simulink model "siasun_config_casadi_VS_lsj_robot_16a"  (R2020a)
settings: Solver=FixedStepAuto  StartTime=0.0  StopTime=inf  FixedStep=0.001  RelTol=1e-3  EnableMultiTasking=on
libraries: Robot_ToolBox x20
(part 1 of 6)
settings Model: SimulationMode=external  Creator=Wang Yifan  LastModifiedBy=admin
settings DataIOCC: ReturnWorkspaceOutputs=off
settings OptimizationCC: LifeSpan=Inf  EfficientTunableParamExpr=on
settings DebuggingCC: SFUnexpectedBacktrackingDiag=warning  SFNoUnconditionalDefaultTransitionDiag=warning  ArithmeticOperatorsInVariantConditions=warning
settings HardwareCC: ProdBitPerLong=64  ProdHWDeviceType=Intel->x86-64 (Linux 64)  TargetBitPerLong=64  TargetBitPerPointer=64  TargetBitPerSizeT=64  TargetBitPerPtrDiffT=64  TargetLargestAtomicFloat=Float  TargetIntDivRoundTo=Zero  TargetEndianess=LittleEndian  TargetWordSize=64  TargetHWDeviceType=Intel->x86-64 (Linux 64)  ProdEqTarget=off
settings SFSimCC: SimUseLocalCustomCode=off  MATLABDynamicMemAlloc=off  CustomCodeUndefinedFunction=UseInterfaceOnly
settings RTWCC: Description=Linux Embedded Real-Time target  SystemTargetFile=linux_ert_target.tlc  GenCodeOnly=on  MakeCommand=make_rtw CC=gcc  TemplateMakefile=linux_ert_target.tmf  RetainRTWFile=on  RTWUseLocalCustomCode=off
settings CodeAppCC: ForceParamTrailComments=on  IgnoreCustomStorageClasses=off  OperatorAnnotations=on  SimulinkDataObjDesc=on  SFDataObjDesc=on  MATLABFcnDesc=on  InsertBlockDesc=on  StateflowObjectComments=on  MATLABSourceComments=on
settings STFCustomTargetCC: CombineOutputUpdateFcns=on  ERTCustomFileBanners=on  SupportContinuousTime=off  SupportNonInlinedSFcns=off  RemoveResetFunc=on  MATLABClassNameForMDSCustomization=Simulink.SoftwareTarget.ERTCustomization  SystemTargetFile=linux_ert_target.tlc
settings ERTTargetCC: MultiwordLength=2048  ParMdlRefBuildCompliant=off  CompOptLevelCompliant=off  ConcurrentExecutionCompliant=off  ModelStepFunctionPrototypeControlCompliant=off  CPPClassGenCompliant=off  UseToolchainInfoCompliant=off  ExtMode=on  ExtModeMexArgs='192.168.0.99' 1 17725  ERTSrcFileBannerTemplate=linux_ert_target_code_template.cgt  ERTHdrFileBannerTemplate=linux_ert_target_code_template.cgt  ERTDataSrcFileTemplate=linux_ert_target_code_template.cgt  ERTDataHdrFileTemplate=linux_ert_target_code_template.cgt  ERTCustomFileTemplate=linux_ert_target_generate_main.tlc
settings ConfigComp: CovMetricSettings=dw  CovSaveCumulativeToWorkspaceVar=on  CovSaveSingleToWorkspaceVar=on  CovExternalEMLEnable=off

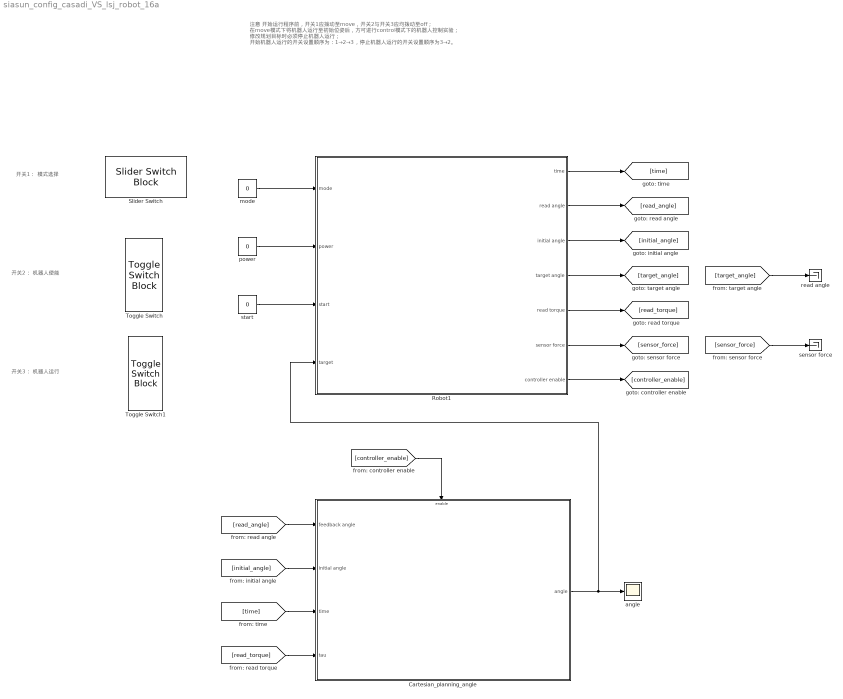
== system siasun_config_casadi_VS_lsj_robot_16a ==
  note: 开关3： 机器人运行
  note: 开关1： 模式选择
  note: 开关2： 机器人使能
  note: 注意
      |
      | 开始运行程序前，开关1应拨动至move，开关2与开关3应均拨动至off；
      | 在move模式下将机器人运行至初始位姿后，方可进行control模式下的机器人控制实验；
      | 修改规划目标时必须停止机器人运行；
      | 开始机器人运行的开关设置顺序为：1→2→3，停止机器人运行的开关设置顺序为3→2。
  Cartesian_planning_angle : Subsystem
  Robot1 : Subsystem  mask{move_joint=[0 0 0 0 0 0], joint_1_limit=[-pi*0.94, pi*0.94], joint_2_limit=[-pi/2, pi*0.72], joint_3_limit=[-pi*0.94, pi*0.42], joint_4_limit=[-pi/1, pi/1], joint_5_limit=[-pi*0.67, pi*0.67], joint_6_limit=[-pi/0.5, pi/0.5]}
      mask prompts: joint_1_limit "Joint 1"; joint_2_limit "Joint 2"; joint_3_limit "Joint 3"; joint_4_limit "Joint 4"; joint_5_limit "Joint 5"; joint_6_limit "Joint 6"
      mask DialogControl Container1 Prompt: 目标关节角(rad)
      mask DialogControl Control1 Prompt: e.g. [0 0 0 0 0 0]
      mask DialogControl Container2 Prompt: 关节限位(rad)
      mask DialogControl Control2 Prompt: e.g. [-pi/2, pi/2]
      mask DialogControl Container3 Prompt: 注意：不需要对此模块内部进行修改
  Slider Switch : SliderSwitchBlock  LabelPosition=Hide
      settings: Values={{'control', 'move'}, [0 1]}
  Toggle Switch : ToggleSwitchBlock  LabelPosition=Hide
      settings: Values={{'Off', 'On'}, [0 1]}
  Toggle Switch1 : ToggleSwitchBlock  LabelPosition=Hide
      settings: Values={{'Off', 'On'}, [0 1]}
  angle : Scope
  mode : Constant  Value=0
  power : Constant  Value=0
  read angle : Terminator
  sensor force : Terminator
  start : Constant  Value=0
  wires:
  mode/1 -> Robot1/1(mode)
  power/1 -> Robot1/2(power)
  Robot1/2(read angle) -> [read_angle]
  Robot1/1(time) -> [time]
  Robot1/7(controller enable) -> [controller_enable]
  Robot1/4(target angle) -> [target_angle]
  Robot1/6(sensor force) -> [sensor_force]
  Robot1/3(initial angle) -> [initial_angle]
  Robot1/5(read torque) -> [read_torque]
  [read_torque] -> Cartesian_planning_angle/4(tau)
  [sensor_force] -> sensor force/1
  start/1 -> Robot1/3(start)
  Cartesian_planning_angle/1(angle) -> angle/1, Robot1/4(target)
  [controller_enable] -> Cartesian_planning_angle/Enable
  [initial_angle] -> Cartesian_planning_angle/2(initial angle)
  [time] -> Cartesian_planning_angle/3(time)
  [read_angle] -> Cartesian_planning_angle/1(feedback angle)
  [target_angle] -> read angle/1

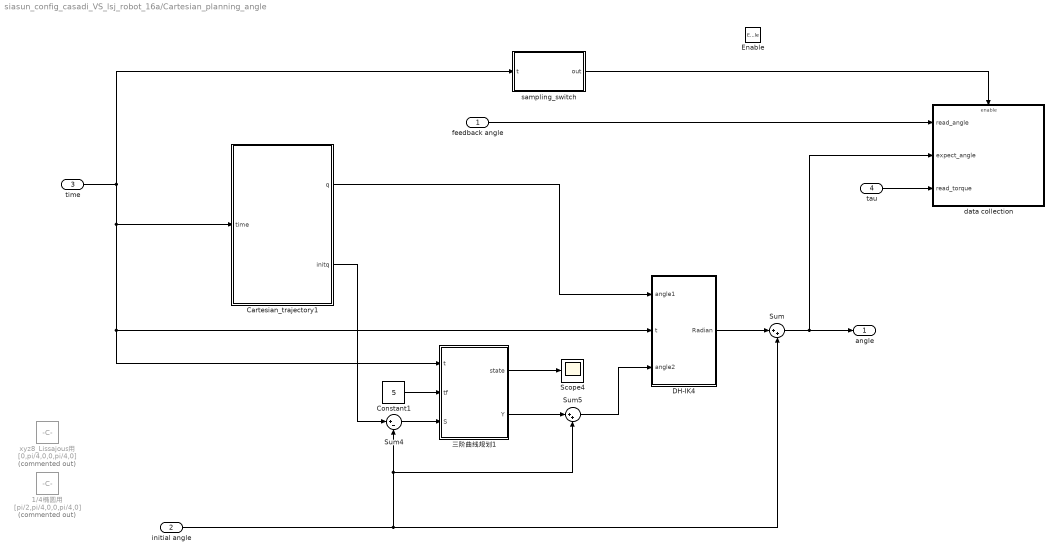
== system siasun_config_casadi_VS_lsj_robot_16a/Cartesian_planning_angle ==
  feedback angle : Inport
  initial angle : Inport  Port=2
  time : Inport  Port=3
  tau : Inport  Port=4
  Enable : EnablePort
  1/4椭圆用 : Constant  Commented=on  Value=[pi/2,pi/4,0,0,pi/4,0]
  Cartesian_trajectory1 : MATLAB Function  TreatAsAtomicUnit=on
  Constant1 : Constant  Value=5
  DH-IK4 : MATLAB Function  TreatAsAtomicUnit=on
  Scope4 : Scope
  Sum : Sum  Inputs=|++
  Sum4 : Sum  Inputs=|+-
  Sum5 : Sum  Inputs=|++
  data collection : Subsystem
  sampling_switch : MATLAB Function  TreatAsAtomicUnit=on
  xyz8_Lissajous用 : Constant  Commented=on  Value=[0,pi/4,0,0,pi/4,0]
  三阶曲线规划1 : Subsystem
  angle : Outport
  wires:
  DH-IK4/1(Radian) -> Sum/1
  Cartesian_trajectory1/1(q) -> DH-IK4/1(angle1)
  initial angle/1 -> Sum5/2, Sum4/2, Sum/2
  Sum4/1 -> 三阶曲线规划1/3(S)
  Constant1/1 -> 三阶曲线规划1/2(tf)
  三阶曲线规划1/1(state) -> Scope4/1
  三阶曲线规划1/2(Y) -> Sum5/1
  Sum5/1 -> DH-IK4/3(angle2)
  sampling_switch/1(out) -> data collection/Enable
  feedback angle/1 -> data collection/1(read_angle)
  Sum/1 -> angle/1, data collection/2(expect_angle)
  time/1 -> DH-IK4/2(t), 三阶曲线规划1/1(t), Cartesian_trajectory1/1(time), sampling_switch/1(t)
  tau/1 -> data collection/3(read_torque)
  Cartesian_trajectory1/2(initq) -> Sum4/1

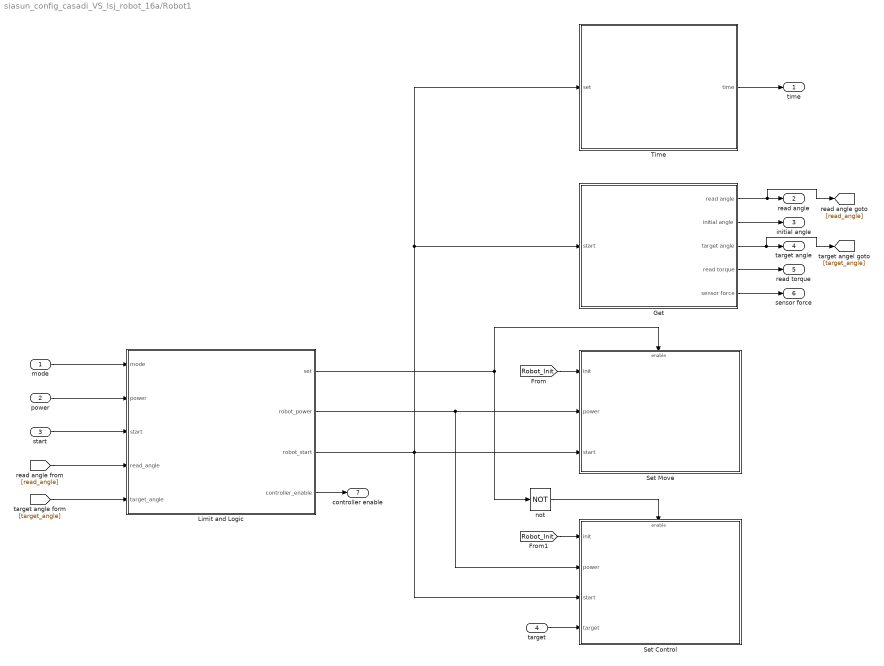
== system siasun_config_casadi_VS_lsj_robot_16a/Robot1 ==
  mode : Inport
  power : Inport  Port=2
  start : Inport  Port=3
  target : Inport  Port=4
  Get : Subsystem
  Limit and Logic : Subsystem
  Set Control : Subsystem  mask(机器人控制模式){mode=Position Mode}
      mask prompts: mode "Control Mode"
      mask TypeOptions mode: Position Mode | Torque Mode | Velocity Mode
  Set Move : Subsystem
  Time : Subsystem
  not : Logic  Operator=NOT  AllPortsSameDT=off  OutDataTypeStr=boolean
  time : Outport
  read angle : Outport  Port=2
  initial angle : Outport  Port=3
  target angle : Outport  Port=4
  read torque : Outport  Port=5
  sensor force : Outport  Port=6
  controller enable : Outport  Port=7
  wires:
  target/1 -> Set Control/4(target)
  Get/1(read angle) -> [read_angle], read angle/1
  Time/1(time) -> time/1
  Get/2(initial angle) -> initial angle/1
  Get/3(target angle) -> [target_angle], target angle/1
  Get/5(sensor force) -> sensor force/1
  Limit and Logic/1(set) -> Set Move/Enable, not/1
  not/1 -> Set Control/Enable
  Limit and Logic/2(robot_power) -> Set Control/2(power), Set Move/2(power)
  Limit and Logic/4(controller_enable) -> controller enable/1
  Limit and Logic/3(robot_start) -> Set Control/3(start), Set Move/3(start), Time/1(set), Get/1(start)
  [Robot_Init] -> Set Move/1(init)
  [Robot_Init] -> Set Control/1(init)
  Get/4(read torque) -> read torque/1
  mode/1 -> Limit and Logic/1(mode)
  power/1 -> Limit and Logic/2(power)
  start/1 -> Limit and Logic/3(start)
  [read_angle] -> Limit and Logic/4(read_angle)
  [target_angle] -> Limit and Logic/5(target_angle)

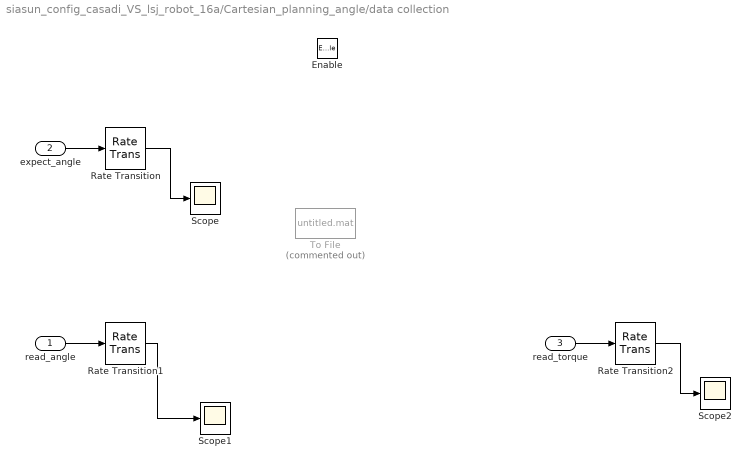
== system siasun_config_casadi_VS_lsj_robot_16a/Cartesian_planning_angle/data collection ==
  read_angle : Inport
  expect_angle : Inport  Port=2
  read_torque : Inport  Port=3
  Enable : EnablePort
  Rate Transition : RateTransition
  Rate Transition1 : RateTransition
  Rate Transition2 : RateTransition
  Scope : Scope
  Scope1 : Scope
  Scope2 : Scope
  To File : ToFile  Commented=on  SaveFormat=Timeseries
  wires:
  Rate Transition/1 -> Scope/1
  Rate Transition1/1 -> Scope1/1
  expect_angle/1 -> Rate Transition/1
  read_angle/1 -> Rate Transition1/1
  Rate Transition2/1 -> Scope2/1
  read_torque/1 -> Rate Transition2/1

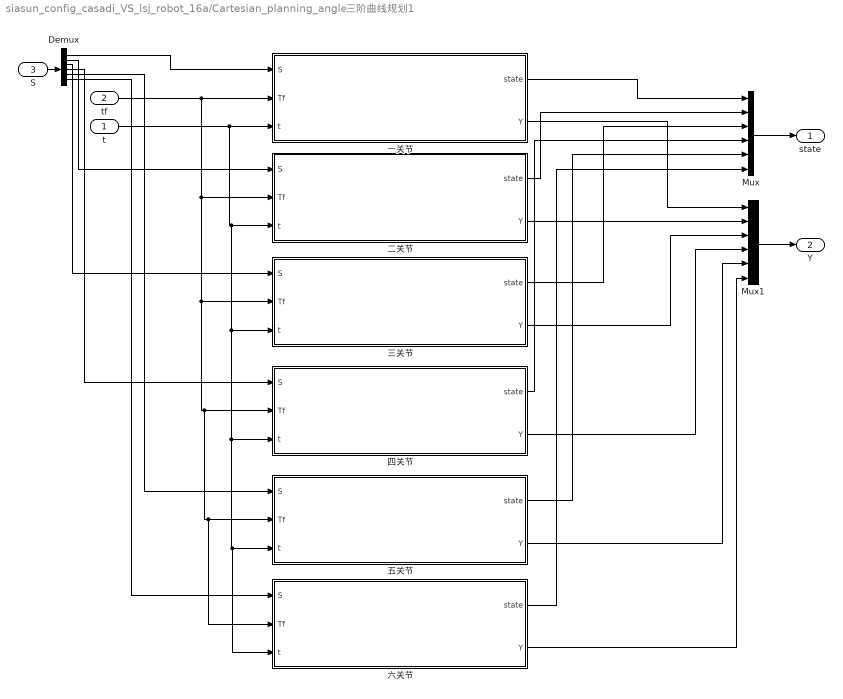
== system siasun_config_casadi_VS_lsj_robot_16a/Cartesian_planning_angle/三阶曲线规划1 ==
  t : Inport
  tf : Inport  Port=2
  S : Inport  Port=3
  Demux : Demux  Outputs=6
  Mux : Mux  Inputs=6
  Mux1 : Mux  Inputs=6
  一关节 : Subsystem
  三关节 : Subsystem
  二关节 : Subsystem
  五关节 : Subsystem
  六关节 : Subsystem
  四关节 : Subsystem
  state : Outport
  Y : Outport  Port=2
  wires:
  一关节/2(Y) -> Mux1/1
  tf/1 -> 六关节/2(Tf), 五关节/2(Tf), 四关节/2(Tf), 三关节/2(Tf), 二关节/2(Tf), 一关节/2(Tf)
  t/1 -> 六关节/3(t), 五关节/3(t), 四关节/3(t), 三关节/3(t), 二关节/3(t), 一关节/3(t)
  一关节/1(state) -> Mux/1
  三关节/1(state) -> Mux/3
  二关节/1(state) -> Mux/2
  四关节/1(state) -> Mux/4
  S/1 -> Demux/1
  Demux/1 -> 一关节/1(S)
  Demux/2 -> 二关节/1(S)
  Demux/3 -> 三关节/1(S)
  Demux/4 -> 四关节/1(S)
  Demux/5 -> 五关节/1(S)
  Demux/6 -> 六关节/1(S)
  Mux1/1 -> Y/1
  二关节/2(Y) -> Mux1/2
  三关节/2(Y) -> Mux1/3
  四关节/2(Y) -> Mux1/4
  五关节/2(Y) -> Mux1/5
  六关节/2(Y) -> Mux1/6
  Mux/1 -> state/1
  五关节/1(state) -> Mux/5
  六关节/1(state) -> Mux/6

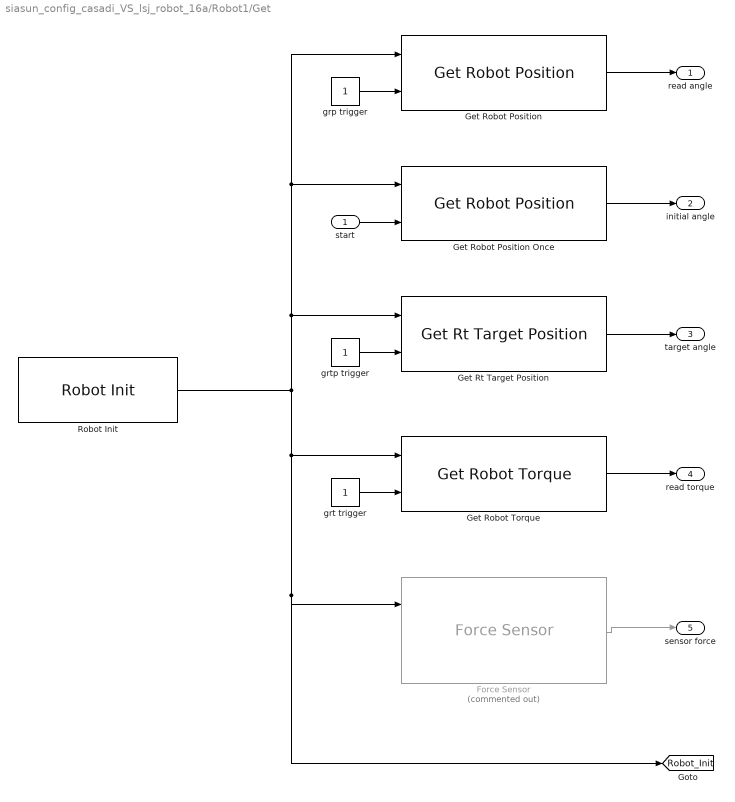
== system siasun_config_casadi_VS_lsj_robot_16a/Robot1/Get ==
  start : Inport
  Force Sensor : Robot_ToolBox/Sensor/Force Sensor  Commented=on  p_robot_index=0  p_torsensor_index=0  p_tool=0  p_wobj=0  p_transform_flag=on
  Get Robot Position : Robot_ToolBox/Robot Interface/Get Robot Position  p_robot_index=0  p_block_index=1  p_read_once=off
  Get Robot Position Once : Robot_ToolBox/Robot Interface/Get Robot Position  p_robot_index=0  p_block_index=0  p_read_once=on
  Get Robot Torque : Robot_ToolBox/Robot Interface/Get Robot Torque  p_robot_index=0  p_block_index=0  p_read_once=off
  Get Rt Target Position : Robot_ToolBox/Robot Interface/Get Rt Target Position  p_robot_index=0  p_block_index=0  p_read_once=off
  Robot Init : Robot_ToolBox/Robot System Tool/Robot Init
  grp trigger : Constant
  grt trigger : Constant
  grtp trigger : Constant
  read angle : Outport
  initial angle : Outport  Port=2
  target angle : Outport  Port=3
  read torque : Outport  Port=4
  sensor force : Outport  Port=5
  tag scope: Robot_Init=global
  wires:
  Robot Init/1 -> Get Robot Position/1, Get Robot Position Once/1, Get Rt Target Position/1, [Robot_Init], Force Sensor/1, Get Robot Torque/1
  Get Robot Position/1 -> read angle/1
  Get Robot Position Once/1 -> initial angle/1
  Get Rt Target Position/1 -> target angle/1
  Force Sensor/1 -> sensor force/1
  grp trigger/1 -> Get Robot Position/2
  grtp trigger/1 -> Get Rt Target Position/2
  start/1 -> Get Robot Position Once/2
  grt trigger/1 -> Get Robot Torque/2
  Get Robot Torque/1 -> read torque/1

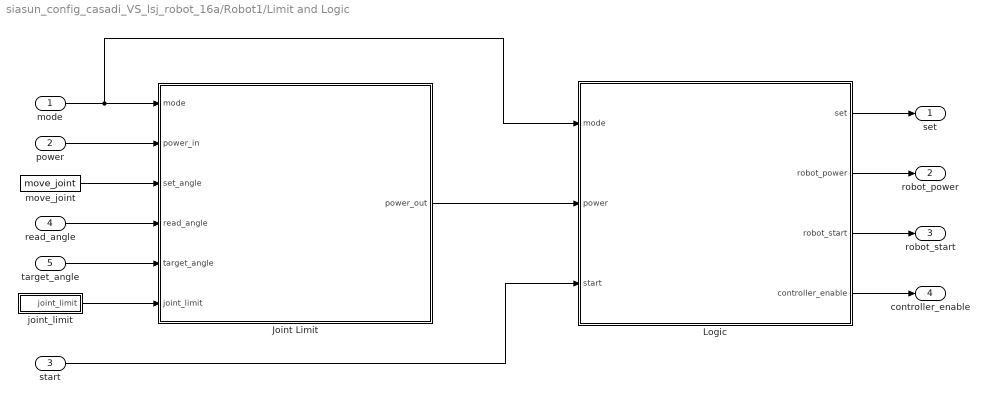
== system siasun_config_casadi_VS_lsj_robot_16a/Robot1/Limit and Logic ==
  mode : Inport
  power : Inport  Port=2
  start : Inport  Port=3
  read_angle : Inport  Port=4
  target_angle : Inport  Port=5
  Joint Limit : MATLAB Function  TreatAsAtomicUnit=on
  Logic : Stateflow chart  TreatAsAtomicUnit=on
  joint_limit : Subsystem
  move_joint : Constant  Value=move_joint
  set : Outport
  robot_power : Outport  Port=2
  robot_start : Outport  Port=3
  controller_enable : Outport  Port=4
  wires:
  Joint Limit/1(power_out) -> Logic/2(power)
  read_angle/1 -> Joint Limit/4(read_angle)
  target_angle/1 -> Joint Limit/5(target_angle)
  mode/1 -> Logic/1(mode), Joint Limit/1(mode)
  power/1 -> Joint Limit/2(power_in)
  start/1 -> Logic/3(start)
  Logic/1(set) -> set/1
  Logic/2(robot_power) -> robot_power/1
  Logic/3(robot_start) -> robot_start/1
  Logic/4(controller_enable) -> controller_enable/1
  move_joint/1 -> Joint Limit/3(set_angle)
  joint_limit/1(joint_limit) -> Joint Limit/6(joint_limit)

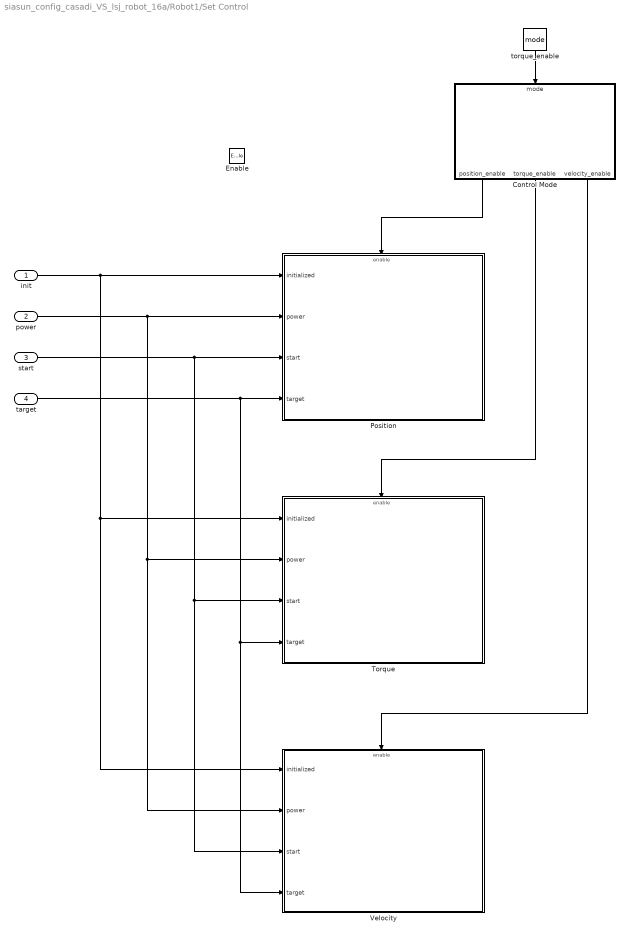
== system siasun_config_casadi_VS_lsj_robot_16a/Robot1/Set Control ==
  init : Inport
  power : Inport  Port=2
  start : Inport  Port=3
  target : Inport  Port=4
  Enable : EnablePort
  Control Mode : Stateflow chart  TreatAsAtomicUnit=on
  Position : Subsystem
  Torque : Subsystem
  Velocity : Subsystem
  torque_enable : Constant  Value=mode
  wires:
  init/1 -> Position/1(initialized), Velocity/1(initialized), Torque/1(initialized)
  power/1 -> Velocity/2(power), Torque/2(power), Position/2(power)
  start/1 -> Velocity/3(start), Torque/3(start), Position/3(start)
  target/1 -> Velocity/4(target), Torque/4(target), Position/4(target)
  Control Mode/1(position_enable) -> Position/Enable
  torque_enable/1 -> Control Mode/1(mode)
  Control Mode/2(torque_enable) -> Torque/Enable
  Control Mode/3(velocity_enable) -> Velocity/Enable

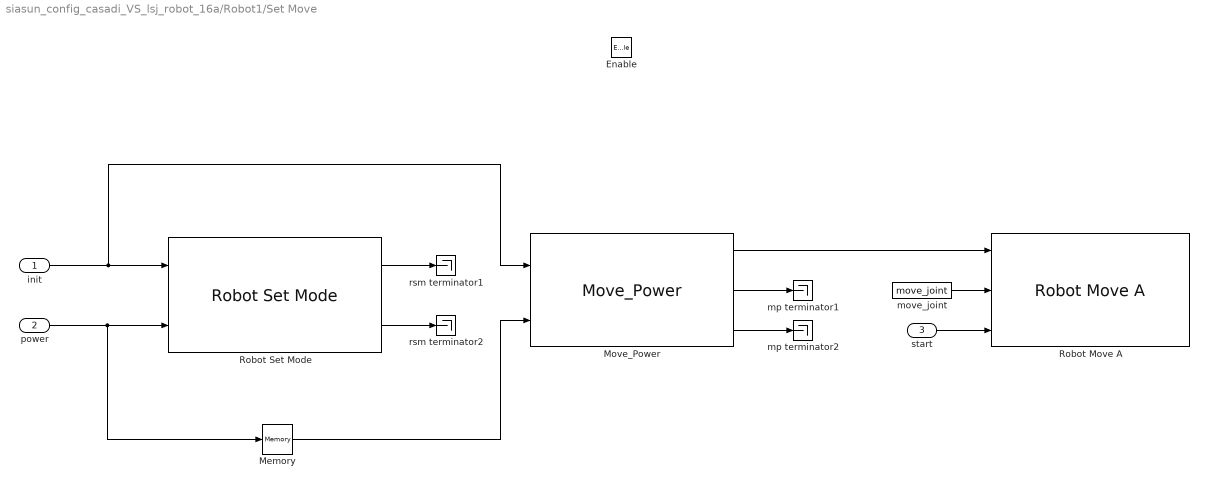
== system siasun_config_casadi_VS_lsj_robot_16a/Robot1/Set Move ==
  init : Inport
  power : Inport  Port=2
  start : Inport  Port=3
  Enable : EnablePort
  Memory : Memory
  Move_Power : Robot_ToolBox/Robot Base Conrtrol/Move_Power  p_robot_index=0  p_block_index=0
      link override S-Function Builder: Parameters=p_robot_index,p_block_index,p_move_thread
  Robot Move A : Robot_ToolBox/Robot Base Conrtrol/Robot Move A  p_robot_index=0  p_block_index=0  p_MoveA_per=[10 10 10 10 10 10]  p_MoveA_per_flag=2  p_zone=0  p_tool=0  p_wobj=0
      link override MoveA: Parameters=p_robot_index,p_block_index,p_MoveA_per,int32(p_MoveA_per_flag),p_zone,p_tool,p_wobj
  Robot Set Mode : Robot_ToolBox/Robot System Tool/Robot Set Mode  p_robot_index=0  p_block_index=0  p_robot_mode=位置模式  p_robot_all=on  p_robot_Axis1=on  p_robot_Axis2=on  p_robot_Axis3=on  p_robot_Axis4=on  p_robot_Axis5=on  p_robot_Axis6=on  p_robot_Axis_add=off
  move_joint : Constant  Value=move_joint
  mp terminator1 : Terminator
  mp terminator2 : Terminator
  rsm terminator1 : Terminator
  rsm terminator2 : Terminator
  wires:
  Move_Power/1 -> Robot Move A/1
  move_joint/1 -> Robot Move A/2
  Move_Power/2 -> mp terminator1/1
  Move_Power/3 -> mp terminator2/1
  start/1 -> Robot Move A/3
  power/1 -> Robot Set Mode/2, Memory/1
  Robot Set Mode/1 -> rsm terminator1/1
  Memory/1 -> Move_Power/2
  Robot Set Mode/2 -> rsm terminator2/1
  init/1 -> Move_Power/1, Robot Set Mode/1

== system siasun_config_casadi_VS_lsj_robot_16a/Robot1/Time ==
  set : Inport
  MATLAB Function : MATLAB Function  TreatAsAtomicUnit=on
  Memory : Memory
  time : Outport
  wires:
  set/1 -> MATLAB Function/1(set)
  MATLAB Function/1(t_out) -> time/1, Memory/1
  Memory/1 -> MATLAB Function/2(t_in)

== system siasun_config_casadi_VS_lsj_robot_16a/Cartesian_planning_angle/三阶曲线规划1/一关节 ==
  S : Inport
  Tf : Inport  Port=2
  t : Inport  Port=3
  3_planning1 : MATLAB Function  TreatAsAtomicUnit=on  mask{g_vs=0, g_ve=0}
      mask prompts: g_vs "初始速度"; g_ve "末速度"
  Interpolation3 : MATLAB Function  TreatAsAtomicUnit=on
  state : Outport
  Y : Outport  Port=2
  wires:
  t/1 -> Interpolation3/4(t)
  S/1 -> 3_planning1/1(S)
  3_planning1/1(state) -> Interpolation3/1(Enable)
  3_planning1/2(plan3_A) -> Interpolation3/2(plan3_A)
  3_planning1/3(tf) -> Interpolation3/3(tf)
  Tf/1 -> 3_planning1/2("tf ")
  Interpolation3/2(Y) -> Y/1
  Interpolation3/1(state) -> state/1

== system siasun_config_casadi_VS_lsj_robot_16a/Cartesian_planning_angle/三阶曲线规划1/三关节 ==
  S : Inport
  Tf : Inport  Port=2
  t : Inport  Port=3
  3_planning1 : MATLAB Function  TreatAsAtomicUnit=on  mask{g_vs=0, g_ve=0}
      mask prompts: g_vs "初始速度"; g_ve "末速度"
  Interpolation3 : MATLAB Function  TreatAsAtomicUnit=on
  state : Outport
  Y : Outport  Port=2
  wires:
  t/1 -> Interpolation3/4(t)
  S/1 -> 3_planning1/1(S)
  3_planning1/1(state) -> Interpolation3/1(Enable)
  3_planning1/2(plan3_A) -> Interpolation3/2(plan3_A)
  3_planning1/3(tf) -> Interpolation3/3(tf)
  Tf/1 -> 3_planning1/2("tf ")
  Interpolation3/2(Y) -> Y/1
  Interpolation3/1(state) -> state/1

== system siasun_config_casadi_VS_lsj_robot_16a/Cartesian_planning_angle/三阶曲线规划1/二关节 ==
  S : Inport
  Tf : Inport  Port=2
  t : Inport  Port=3
  3_planning1 : MATLAB Function  TreatAsAtomicUnit=on  mask{g_vs=0, g_ve=0}
      mask prompts: g_vs "初始速度"; g_ve "末速度"
  Interpolation3 : MATLAB Function  TreatAsAtomicUnit=on
  state : Outport
  Y : Outport  Port=2
  wires:
  t/1 -> Interpolation3/4(t)
  S/1 -> 3_planning1/1(S)
  3_planning1/1(state) -> Interpolation3/1(Enable)
  3_planning1/2(plan3_A) -> Interpolation3/2(plan3_A)
  3_planning1/3(tf) -> Interpolation3/3(tf)
  Tf/1 -> 3_planning1/2("tf ")
  Interpolation3/2(Y) -> Y/1
  Interpolation3/1(state) -> state/1

== system siasun_config_casadi_VS_lsj_robot_16a/Cartesian_planning_angle/三阶曲线规划1/五关节 ==
  S : Inport
  Tf : Inport  Port=2
  t : Inport  Port=3
  3_planning1 : MATLAB Function  TreatAsAtomicUnit=on  mask{g_vs=0, g_ve=0}
      mask prompts: g_vs "初始速度"; g_ve "末速度"
  Interpolation3 : MATLAB Function  TreatAsAtomicUnit=on
  state : Outport
  Y : Outport  Port=2
  wires:
  t/1 -> Interpolation3/4(t)
  S/1 -> 3_planning1/1(S)
  3_planning1/1(state) -> Interpolation3/1(Enable)
  3_planning1/2(plan3_A) -> Interpolation3/2(plan3_A)
  3_planning1/3(tf) -> Interpolation3/3(tf)
  Tf/1 -> 3_planning1/2("tf ")
  Interpolation3/2(Y) -> Y/1
  Interpolation3/1(state) -> state/1

== system siasun_config_casadi_VS_lsj_robot_16a/Cartesian_planning_angle/三阶曲线规划1/六关节 ==
  S : Inport
  Tf : Inport  Port=2
  t : Inport  Port=3
  3_planning1 : MATLAB Function  TreatAsAtomicUnit=on  mask{g_vs=0, g_ve=0}
      mask prompts: g_vs "初始速度"; g_ve "末速度"
  Interpolation3 : MATLAB Function  TreatAsAtomicUnit=on
  state : Outport
  Y : Outport  Port=2
  wires:
  t/1 -> Interpolation3/4(t)
  S/1 -> 3_planning1/1(S)
  3_planning1/1(state) -> Interpolation3/1(Enable)
  3_planning1/2(plan3_A) -> Interpolation3/2(plan3_A)
  3_planning1/3(tf) -> Interpolation3/3(tf)
  Tf/1 -> 3_planning1/2("tf ")
  Interpolation3/2(Y) -> Y/1
  Interpolation3/1(state) -> state/1

== system siasun_config_casadi_VS_lsj_robot_16a/Cartesian_planning_angle/三阶曲线规划1/四关节 ==
  S : Inport
  Tf : Inport  Port=2
  t : Inport  Port=3
  3_planning1 : MATLAB Function  TreatAsAtomicUnit=on  mask{g_vs=0, g_ve=0}
      mask prompts: g_vs "初始速度"; g_ve "末速度"
  Interpolation3 : MATLAB Function  TreatAsAtomicUnit=on
  state : Outport
  Y : Outport  Port=2
  wires:
  t/1 -> Interpolation3/4(t)
  S/1 -> 3_planning1/1(S)
  3_planning1/1(state) -> Interpolation3/1(Enable)
  3_planning1/2(plan3_A) -> Interpolation3/2(plan3_A)
  3_planning1/3(tf) -> Interpolation3/3(tf)
  Tf/1 -> 3_planning1/2("tf ")
  Interpolation3/2(Y) -> Y/1
  Interpolation3/1(state) -> state/1

== system siasun_config_casadi_VS_lsj_robot_16a/Robot1/Limit and Logic/joint_limit ==
  Mux : Mux  Inputs=6
  c1 : Constant  Value=joint_1_limit
  c2 : Constant  Value=joint_2_limit
  c3 : Constant  Value=joint_3_limit
  c4 : Constant  Value=joint_4_limit
  c5 : Constant  Value=joint_5_limit
  c6 : Constant  Value=joint_6_limit
  joint_limit : Outport
  wires:
  c1/1 -> Mux/1
  c2/1 -> Mux/2
  c3/1 -> Mux/3
  c4/1 -> Mux/4
  c5/1 -> Mux/5
  c6/1 -> Mux/6
  Mux/1 -> joint_limit/1

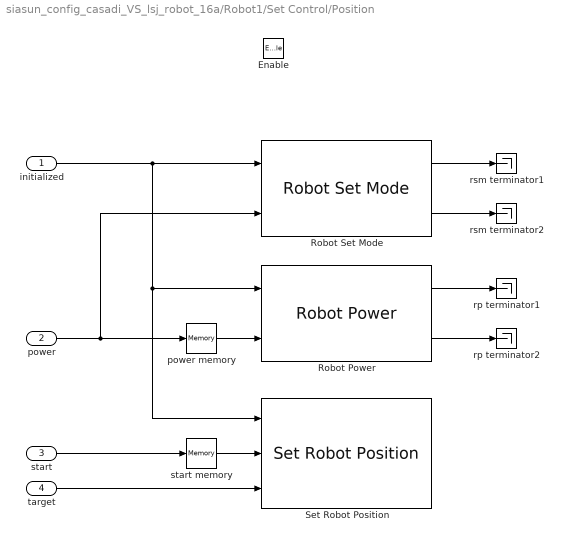
== system siasun_config_casadi_VS_lsj_robot_16a/Robot1/Set Control/Position ==
  initialized : Inport
  power : Inport  Port=2
  start : Inport  Port=3
  target : Inport  Port=4
  Enable : EnablePort
  Robot Power : Robot_ToolBox/Robot System Tool/Robot Power  p_robot_index=0  p_block_index=0  p_robot_all=on  p_robot_Axis1=on  p_robot_Axis2=on  p_robot_Axis3=on  p_robot_Axis4=on  p_robot_Axis5=on  p_robot_Axis6=on  p_robot_Axis_add=off
  Robot Set Mode : Robot_ToolBox/Robot System Tool/Robot Set Mode  p_robot_index=0  p_block_index=0  p_robot_mode=位置模式  p_robot_all=on  p_robot_Axis1=on  p_robot_Axis2=on  p_robot_Axis3=on  p_robot_Axis4=on  p_robot_Axis5=on  p_robot_Axis6=on  p_robot_Axis_add=off
  Set Robot Position : Robot_ToolBox/Robot Interface/Set Robot Position  p_robot_index=0  p_block_index=0  p_read_once=off
  power memory : Memory
  rp terminator1 : Terminator
  rp terminator2 : Terminator
  rsm terminator1 : Terminator
  rsm terminator2 : Terminator
  start memory : Memory
  wires:
  Robot Set Mode/1 -> rsm terminator1/1
  Robot Set Mode/2 -> rsm terminator2/1
  Robot Power/2 -> rp terminator2/1
  initialized/1 -> Robot Set Mode/1, Robot Power/1, Set Robot Position/1
  target/1 -> Set Robot Position/3
  Robot Power/1 -> rp terminator1/1
  power/1 -> power memory/1, Robot Set Mode/2
  start memory/1 -> Set Robot Position/2
  start/1 -> start memory/1
  power memory/1 -> Robot Power/2

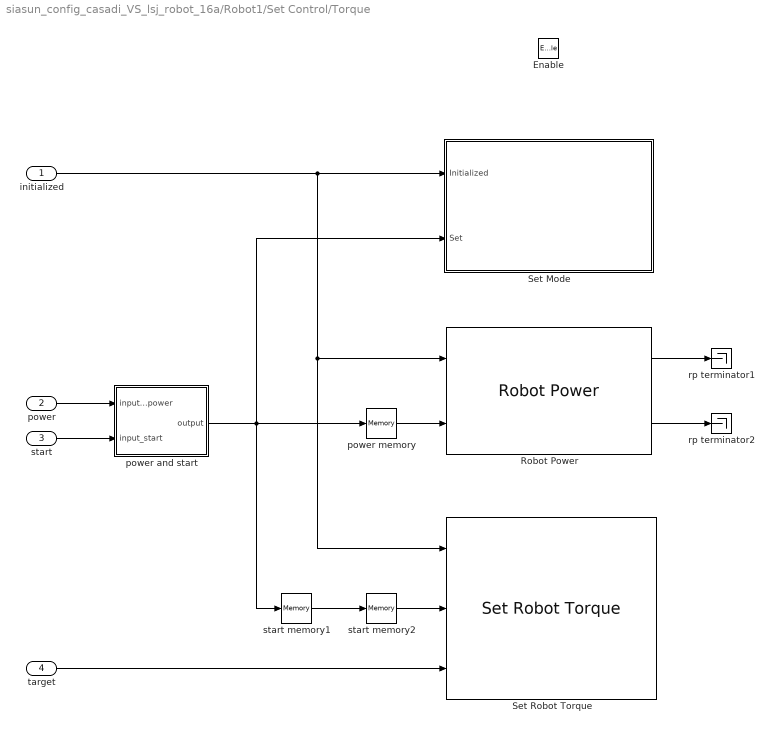
== system siasun_config_casadi_VS_lsj_robot_16a/Robot1/Set Control/Torque ==
  initialized : Inport
  power : Inport  Port=2
  start : Inport  Port=3
  target : Inport  Port=4
  Enable : EnablePort
  Robot Power : Robot_ToolBox/Robot System Tool/Robot Power  p_robot_index=0  p_block_index=0  p_robot_all=off  p_robot_Axis1=off  p_robot_Axis2=off  p_robot_Axis3=off  p_robot_Axis4=off  p_robot_Axis5=off  p_robot_Axis6=on  p_robot_Axis_add=off
  Set Mode : Subsystem
  Set Robot Torque : Robot_ToolBox/Robot Interface/Set Robot Torque  p_robot_index=0  p_block_index=0  p_read_once=off
      link override Set Robot Torque: Parameters=p_robot_index,p_block_index,p_read_once
  power and start : MATLAB Function  TreatAsAtomicUnit=on
  power memory : Memory
  rp terminator1 : Terminator
  rp terminator2 : Terminator
  start memory1 : Memory
  start memory2 : Memory
  wires:
  target/1 -> Set Robot Torque/3
  start memory1/1 -> start memory2/1
  Robot Power/2 -> rp terminator2/1
  Robot Power/1 -> rp terminator1/1
  start memory2/1 -> Set Robot Torque/2
  power memory/1 -> Robot Power/2
  power/1 -> power and start/1(input_power)
  start/1 -> power and start/2(input_start)
  power and start/1(output) -> start memory1/1, Set Mode/2(Set), power memory/1
  initialized/1 -> Robot Power/1, Set Robot Torque/1, Set Mode/1(Initialized)

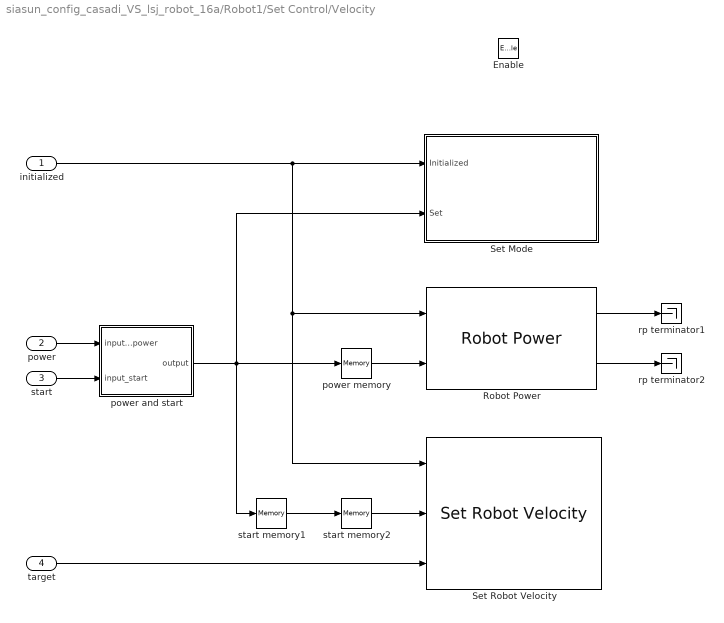
== system siasun_config_casadi_VS_lsj_robot_16a/Robot1/Set Control/Velocity ==
  initialized : Inport
  power : Inport  Port=2
  start : Inport  Port=3
  target : Inport  Port=4
  Enable : EnablePort
  Robot Power : Robot_ToolBox/Robot System Tool/Robot Power  p_robot_index=0  p_block_index=0  p_robot_all=on  p_robot_Axis1=on  p_robot_Axis2=on  p_robot_Axis3=on  p_robot_Axis4=on  p_robot_Axis5=on  p_robot_Axis6=on  p_robot_Axis_add=off
  Set Mode : Subsystem
  Set Robot Velocity : Robot_ToolBox/Robot Interface/Set Robot Velocity  p_robot_index=0  p_block_index=0  p_read_once=off
  power and start : MATLAB Function  TreatAsAtomicUnit=on
  power memory : Memory
  rp terminator1 : Terminator
  rp terminator2 : Terminator
  start memory1 : Memory
  start memory2 : Memory
  wires:
  start memory1/1 -> start memory2/1
  Robot Power/2 -> rp terminator2/1
  Robot Power/1 -> rp terminator1/1
  initialized/1 -> Set Mode/1(Initialized), Robot Power/1, Set Robot Velocity/1
  start memory2/1 -> Set Robot Velocity/2
  power memory/1 -> Robot Power/2
  target/1 -> Set Robot Velocity/3
  power/1 -> power and start/1(input_power)
  start/1 -> power and start/2(input_start)
  power and start/1(output) -> Set Mode/2(Set), power memory/1, start memory1/1

== system siasun_config_casadi_VS_lsj_robot_16a/Robot1/Set Control/Torque/Set Mode ==
  Initialized : Inport
  Set : Inport  Port=2
  Not : MATLAB Function  TreatAsAtomicUnit=on
  Set Position Mode : Subsystem
  Set Torque Mode : Subsystem
  wires:
  Initialized/1 -> Set Position Mode/1(Initialized), Set Torque Mode/1(Initialized)
  Set/1 -> Set Torque Mode/2(Set), Not/1(in)
  Not/1(out) -> Set Position Mode/2(Set)

== system siasun_config_casadi_VS_lsj_robot_16a/Robot1/Set Control/Velocity/Set Mode ==
  Initialized : Inport
  Set : Inport  Port=2
  Not : MATLAB Function  TreatAsAtomicUnit=on
  Set Position Mode : Subsystem
  Set Velocity Mode : Subsystem
  wires:
  Initialized/1 -> Set Position Mode/1(Initialitzed), Set Velocity Mode/1(Initialitzed)
  Set/1 -> Set Velocity Mode/2(Set), Not/1(in)
  Not/1(out) -> Set Position Mode/2(Set)

== system siasun_config_casadi_VS_lsj_robot_16a/Robot1/Set Control/Torque/Set Mode/Set Position Mode ==
  Initialized : Inport
  Set : Inport  Port=2
  Robot Set Mode : Robot_ToolBox/Robot System Tool/Robot Set Mode  p_robot_index=0  p_block_index=0  p_robot_mode=位置模式  p_robot_all=on  p_robot_Axis1=on  p_robot_Axis2=on  p_robot_Axis3=on  p_robot_Axis4=on  p_robot_Axis5=on  p_robot_Axis6=on  p_robot_Axis_add=off
  rsm terminator1 : Terminator
  rsm terminator2 : Terminator
  wires:
  Initialized/1 -> Robot Set Mode/1
  Robot Set Mode/1 -> rsm terminator1/1
  Robot Set Mode/2 -> rsm terminator2/1
  Set/1 -> Robot Set Mode/2

== system siasun_config_casadi_VS_lsj_robot_16a/Robot1/Set Control/Torque/Set Mode/Set Torque Mode ==
  Initialized : Inport
  Set : Inport  Port=2
  Robot Set Mode : Robot_ToolBox/Robot System Tool/Robot Set Mode  p_robot_index=0  p_block_index=0  p_robot_mode=力矩模式  p_robot_all=on  p_robot_Axis1=on  p_robot_Axis2=on  p_robot_Axis3=on  p_robot_Axis4=on  p_robot_Axis5=on  p_robot_Axis6=on  p_robot_Axis_add=off
  rsm terminator1 : Terminator
  rsm terminator2 : Terminator
  wires:
  Robot Set Mode/2 -> rsm terminator2/1
  Robot Set Mode/1 -> rsm terminator1/1
  Set/1 -> Robot Set Mode/2
  Initialized/1 -> Robot Set Mode/1

== system siasun_config_casadi_VS_lsj_robot_16a/Robot1/Set Control/Velocity/Set Mode/Set Position Mode ==
  Initialitzed : Inport
  Set : Inport  Port=2
  Robot Set Mode : Robot_ToolBox/Robot System Tool/Robot Set Mode  p_robot_index=0  p_block_index=0  p_robot_mode=位置模式  p_robot_all=on  p_robot_Axis1=on  p_robot_Axis2=on  p_robot_Axis3=on  p_robot_Axis4=on  p_robot_Axis5=on  p_robot_Axis6=on  p_robot_Axis_add=off
  rsm terminator1 : Terminator
  rsm terminator2 : Terminator
  wires:
  Robot Set Mode/1 -> rsm terminator1/1
  Robot Set Mode/2 -> rsm terminator2/1
  Initialitzed/1 -> Robot Set Mode/1
  Set/1 -> Robot Set Mode/2

== system siasun_config_casadi_VS_lsj_robot_16a/Robot1/Set Control/Velocity/Set Mode/Set Velocity Mode ==
  Initialitzed : Inport
  Set : Inport  Port=2
  Robot Set Mode : Robot_ToolBox/Robot System Tool/Robot Set Mode  p_robot_index=0  p_block_index=0  p_robot_mode=速度模式  p_robot_all=on  p_robot_Axis1=on  p_robot_Axis2=on  p_robot_Axis3=on  p_robot_Axis4=on  p_robot_Axis5=on  p_robot_Axis6=on  p_robot_Axis_add=off
  rsm terminator1 : Terminator
  rsm terminator2 : Terminator
  wires:
  Robot Set Mode/1 -> rsm terminator1/1
  Robot Set Mode/2 -> rsm terminator2/1
  Initialitzed/1 -> Robot Set Mode/1
  Set/1 -> Robot Set Mode/2

== stateflow chart siasun_config_casadi_VS_lsj_robot_16a/Robot1/Limit and Logic/Logic ==
  state init
    entry:
    robot_power = 0;
    robot_start = 0;
    controller_enable = 0;
  state move
    entry: set = 1;
    state move_power_on
      entry: robot_power = 1;
      state robot_start_on
        entry:
        robot_start = 1;
        controller_enable = 0;
      state robot_start_off
        entry:
        robot_start = 0;
        controller_enable = 0;
      (default) -> (junction 90)
      (junction 90) -> move.move_power_on.robot_start_off [order 2] : [start == 0]
      (junction 90) -> move.move_power_on.robot_start_on [order 1] : [start == 1]
      move.move_power_on.robot_start_on -> move.move_power_on.robot_start_off : [start == 0]
      move.move_power_on.robot_start_off -> move.move_power_on.robot_start_on : [start == 1]
    state move_power_off
      entry: robot_power = 0;
      state robot_start_off
        entry:
        robot_start = 0;
        controller_enable = 0;
      (default) -> move.move_power_off.robot_start_off
    (default) -> (junction 40)
    (junction 40) -> move_power_off [order 2] : [power == 0]
    (junction 40) -> move_power_on [order 1] : [power == 1]
    move_power_on -> move_power_off : [power == 0]
    move_power_off -> move_power_on : [power == 1 & start == 0]
  state control
    entry: set = 0;
    state control_power_on
      entry: robot_power = 1;
      state robot_start_off
        entry:
        robot_start = 0;
        controller_enable = 0;
      state robot_start_on
        entry:
        robot_start = 1;
        controller_enable = 1;
      (default) -> (junction 73)
      (junction 73) -> control.control_power_on.robot_start_on [order 1] : [start == 1]
      (junction 73) -> control.control_power_on.robot_start_off [order 2] : [start == 0]
      control.control_power_on.robot_start_on -> control.control_power_on.robot_start_off : [start == 0]
      control.control_power_on.robot_start_off -> control.control_power_on.robot_start_on : [start == 1]
    state control_power_off
      entry: robot_power = 0;
      state robot_start_off
        entry:
        robot_start = 0;
        controller_enable = 0;
      (default) -> control.control_power_off.robot_start_off
    (default) -> (junction 50)
    (junction 50) -> control_power_on [order 1] : [power == 1]
    (junction 50) -> control_power_off [order 2] : [power == 0]
    control_power_on -> control_power_off : [power == 0]
    control_power_off -> control_power_on : [power == 1 & start == 0]
  (default) -> (junction 81)
  (junction 81) -> init [order 2] : [power == 1 | start ==1]
  init -> (junction 81)
  (junction 81) -> (junction 32) [order 1] : [power == 0 & start ==0]
  (junction 32) -> control [order 2] : [mode == 0]
  (junction 32) -> move [order 1] : [mode == 1]
  move -> control : [mode == 0 & power == 0]
  control -> move : [mode == 1 & power == 0]
  data: mode input; power input; start input; set output; robot_power output; robot_start output; controller_enable output

== stateflow chart siasun_config_casadi_VS_lsj_robot_16a/Robot1/Set Control/Control Mode ==
  state Init
    entry:
    position_enable = 1;
    torque_enable = 0;
    velocity_enable = 0;
  state Position
    entry:
    position_enable = 1;
    torque_enable = 0;
    velocity_enable = 0;
  state Torque
    entry:
    position_enable = 0;
    torque_enable = 1;
    velocity_enable = 0;
  state Velocity
    entry:
    position_enable = 0;
    torque_enable = 0;
    velocity_enable = 1;
  (default) -> Init
  Init -> (junction 6)
  (junction 6) -> Velocity [order 3] : [mode == 3]
  (junction 6) -> Position [order 1] : [mode == 1]
  (junction 6) -> Torque [order 2] : [mode == 2]
  data: mode input; position_enable output; torque_enable output; velocity_enable output
